simulink model "actuator"  (R2014a)
settings: Solver=ode45  SolverName=ode3  SolverMode=SingleTasking  StartTime=start_time  StopTime=stop_time  FixedStep=min_step  RelTol=1e-3
undefined symbols (not defined in the file): alpha, amp, c, delta_t, g, initial_disp, initial_velocity, k, m, switchF, target_t
libraries: simulink x1, fuzblock x1
settings Model: CovMetricSettings=dwe  CovHtmlReporting=off  covSaveCumulativeToWorkspaceVar=off  CovSaveSingleToWorkspaceVar=off  CovExternalEMLEnable=on  CovSFcnEnable=on  Creator=mehrab  LastModifiedBy=mehrab
settings DataIOCC: LimitDataPoints=off  SaveFormat=StructureWithTime
settings DebuggingCC: MergeDetectMultiDrivingBlocksExec=error  SolverPrmCheckMsg=none  FrameProcessingCompatibilityMsg=error  SFUnexpectedBacktrackingDiag=error  SFNoUnconditionalDefaultTransitionDiag=error
settings HardwareCC: ProdBitPerPointer=64  ProdLargestAtomicFloat=Float  ProdIntDivRoundTo=Zero  ProdEndianess=LittleEndian  ProdHWDeviceType=Specified
settings ModelReferenceCC: PropagateSignalLabelsOutOfModel=on
settings GRTTargetCC: TargetLangStandard=C99 (ISO)

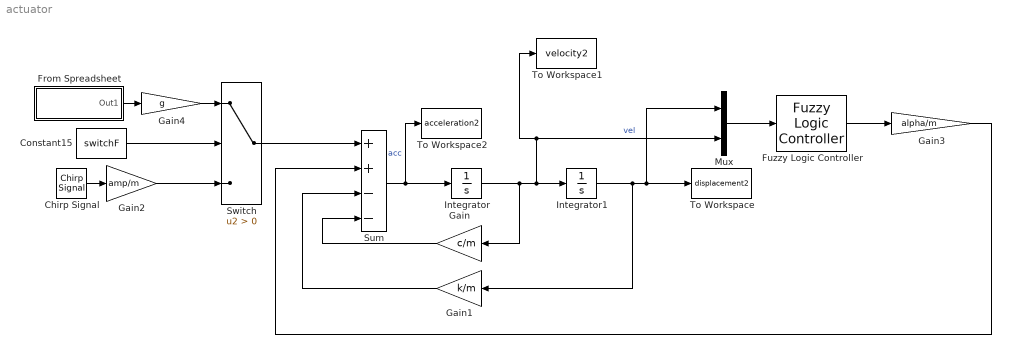
== system actuator ==
  Chirp Signal : simulink/Sources/Chirp Signal  f1=initial_freq  T=target_t  f2=freq_target
  Constant15 : Constant  Value=switchF
  From Spreadsheet : Subsystem  Description=Replaced Block  mask(Replaced Block){}
      mask help: This block has been replaced with an empty subsystem because it used functionality that is unavailable in Simulink R2014a.
      mask Display: fprintf('Replaced: %s\n','FromSpreadsheet')
  Fuzzy Logic Controller : fuzblock/Fuzzy Logic  Controller  FIS='actuatorfuzzy'
  Gain : Gain  Gain=c/m
  Gain1 : Gain  Gain=k/m
  Gain2 : Gain  Gain=amp/m
  Gain3 : Gain  Gain=alpha/m
  Gain4 : Gain  Gain=g
  Integrator : Integrator  InitialCondition=initial_velocity
  Integrator1 : Integrator  InitialCondition=initial_disp
  Mux : Mux  Inputs=2
  Sum : Sum  Inputs=++--
  Switch : Switch  Criteria=u2 > Threshold
  To Workspace : ToWorkspace  VariableName=displacement2  SampleTime=delta_t
  To Workspace1 : ToWorkspace  VariableName=velocity2  SampleTime=delta_t
  To Workspace2 : ToWorkspace  VariableName=acceleration2  SampleTime=delta_t
  wires:
  Chirp Signal/1 -> Gain2/1
  Sum/1 -> To Workspace2/1, Integrator/1  "acc"
  Integrator/1 -> To Workspace1/1, Mux/2, Integrator1/1, Gain/1  "vel"
  Gain/1 -> Sum/4
  Gain1/1 -> Sum/3
  Mux/1 -> Fuzzy Logic Controller/1
  Integrator1/1 -> Mux/1, To Workspace/1, Gain1/1
  Switch/1 -> Sum/1
  Gain2/1 -> Switch/3
  Constant15/1 -> Switch/2
  Gain4/1 -> Switch/1
  From Spreadsheet/1(Out1) -> Gain4/1
  Fuzzy Logic Controller/1 -> Gain3/1
  Gain3/1 -> Sum/2

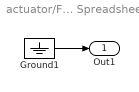
== system actuator/From Spreadsheet ==
  Ground1 : Ground
  Out1 : Outport
  wires:
  Ground1/1 -> Out1/1
